simulink model "cst_robotarm_new"  (R2020a)
settings: Solver=ode23t  StartTime=0.0  StopTime=40  FixedStep=0.0001  MaxStep=0.05  RelTol=1e-3  EnableMultiTasking=on
model workspace (MAT data in the model file):
  DCMotor_J = 0.0946866703633
  DCMotor_K = 0.477771340295
  DCMotor_Kf = 0.921434142151
  DCMotor_L = 0.000316454712175
  DCMotor_R = 4.99938152603
  Ts = 0.1
  dFilt = [1 -0.1202]
  nFilt = [0.4399 0.4399]
undefined symbols (not defined in the file): X, Y, Z
libraries: sm_lib x244, fl_lib x75, nesl_utility x28, ee_lib x21
(part 1 of 6)
settings Model: SimulationMode=accelerator  Creator=The MathWorks, Inc.  LastModifiedBy=nikhil
settings DataIOCC: LimitDataPoints=on  SaveFormat=Array  InspectSignalLogs=on  SaveTime=off  ReturnWorkspaceOutputs=off
settings OptimizationCC: ExpressionDepthLimit=2147483647  LifeSpan=inf
settings DebuggingCC: UnderspecifiedInitializationDetection=Classic  MergeDetectMultiDrivingBlocksExec=none  FcnCallInpInsideContextMsg=warning  StateNameClashWarn=warning  SFUnexpectedBacktrackingDiag=warning  SFNoUnconditionalDefaultTransitionDiag=warning  SFExecutionAtInitializationDiag=none  ArithmeticOperatorsInVariantConditions=warning
settings HardwareCC: ProdBitPerPointer=32  ProdBitPerSizeT=32  ProdBitPerPtrDiffT=32  ProdLargestAtomicFloat=None  ProdIntDivRoundTo=Undefined  ProdEndianess=Unspecified  ProdWordSize=32  ProdHWDeviceType=32-bit Generic
settings ModelReferenceCC: PropagateSignalLabelsOutOfModel=off
settings SFSimCC: SimUseLocalCustomCode=off  CustomCodeUndefinedFunction=UseInterfaceOnly
settings RTWCC: RTWUseLocalCustomCode=off
settings CodeAppCC: StateflowObjectComments=on
settings GRTTargetCC: TargetLangStandard=C89/C90 (ANSI)  CombineOutputUpdateFcns=off  GRTInterface=on
settings ConfigComp: CovMetricSettings=dw  CovHtmlReporting=on  CovSaveCumulativeToWorkspaceVar=on  CovSaveSingleToWorkspaceVar=on  CovExternalEMLEnable=off  CovSFcnEnable=off
settings SimscapeCC: SimscapeNormalizeSystem=off
settings ConfigurationSet: Description=SimMechanics 2G
settings DiagnosticsConfigSet: SimMechanicsUnconnectedFramePorts=none
settings ExplorerConfigSet: SimMechanicsOpenEditorOnUpdate=off  InternalSimMechanicsExplorerSettings="<ExplorerConfiguration><canonicalview>planar_xy</canonicalview><AnimationSetting><BasePlaybackSpeed>1.0</BasePlaybackSpeed><PlaybackSpeedFactor>1.0</PlaybackSpeedFactor></AnimationSetting><TilePanel><TileInfo><Tiles Columns=\"1\" Count=\"1\" Rows=\"1\"><Column Left=\"2\" Weight=\"1\"/><Column Left=\"708\"/><Row Top=\"2\" Weight=\"1\"/><Row Top=\"595\"/><Tile Height=\"1\" Width=\"1\" X=\"0\" Y=\"0\"/></Tiles></TileInfo><SceneInfo><SceneViewer><BGColor><R>0.80000001192092896</R><G>0.80000001192092896</G><B>0.80000001192092896</B></BGColor><Camera><Position><X>0.30752487944302698</X><Y>0.57922836563106395</Y><Z>0.35651305744246536</Z></Position><Center><X>-0.033772386749033274</X><Y>0.23793109943898419</Y><Z>0.015215791250393121</Z></Center><Up><X>-0.40824829046386307</X><Y>0.81649658092772615</Y><Z>-0.40824829046386307</Z></Up><Left>-0.063283674940751766</Left><Right>0.063283674940751766</Right><Bottom>-0.22321517040744418</Bottom><Top>0.22321517040744418</Top></Camera></SceneViewer></SceneInfo></TilePanel></ExplorerConfiguration>"

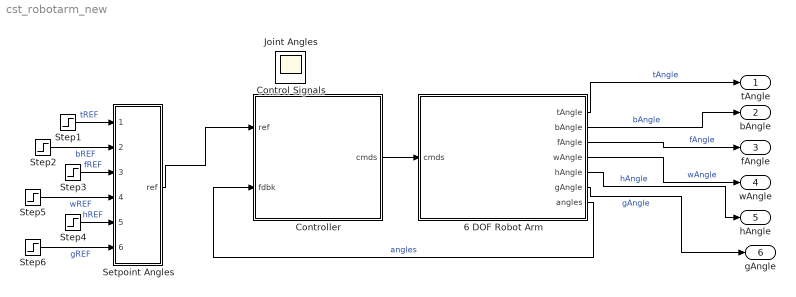
== system cst_robotarm_new ==
  6 DOF Robot Arm : Subsystem
      mask Display: image('RobotArmSystem.jpg',[0.2 0.05 0.6 0.9])
  Controller : Subsystem
  Setpoint Angles : Subsystem
  Step1 : Step  Time=0  After=60  SampleTime=Ts
  Step2 : Step  Time=0  Before=90  After=80  SampleTime=Ts
  Step3 : Step  Time=0  After=60  SampleTime=Ts
  Step4 : Step  Time=0  After=90  SampleTime=Ts
  Step5 : Step  Time=0  After=90  SampleTime=Ts
  Step6 : Step  Time=0  After=60  SampleTime=Ts
  tAngle : Outport
  bAngle : Outport  Port=2
  fAngle : Outport  Port=3
  wAngle : Outport  Port=4
  hAngle : Outport  Port=5
  gAngle : Outport  Port=6
  Control Signals : Scope
  Joint Angles : Scope
  wires:
  Controller/1(cmds) -> 6 DOF Robot Arm/1(cmds)
  6 DOF Robot Arm/7(angles) -> Controller/2(fdbk)  "angles"
  Setpoint Angles/1(ref) -> Controller/1(ref)
  Step2/1 -> Setpoint Angles/2(bREF)  "bREF"
  Step1/1 -> Setpoint Angles/1(tREF)  "tREF"
  Step4/1 -> Setpoint Angles/5(hREF)  "hREF"
  Step5/1 -> Setpoint Angles/4(wREF)  "wREF"
  Step3/1 -> Setpoint Angles/3(fREF)  "fREF"
  Step6/1 -> Setpoint Angles/6(gREF)  "gREF"
  6 DOF Robot Arm/1(tAngle) -> tAngle/1  "tAngle"
  6 DOF Robot Arm/2(bAngle) -> bAngle/1  "bAngle"
  6 DOF Robot Arm/3(fAngle) -> fAngle/1  "fAngle"
  6 DOF Robot Arm/4(wAngle) -> wAngle/1  "wAngle"
  6 DOF Robot Arm/5(hAngle) -> hAngle/1  "hAngle"
  6 DOF Robot Arm/6(gAngle) -> gAngle/1  "gAngle"

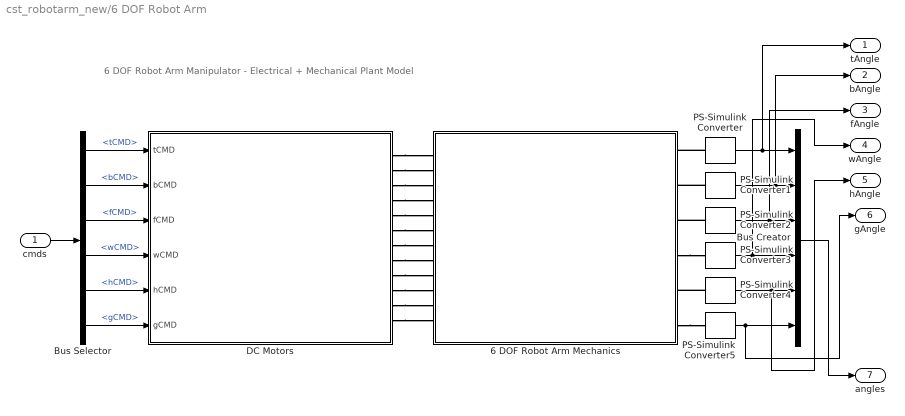
== system cst_robotarm_new/6 DOF Robot Arm ==
  note: 6 DOF Robot Arm Manipulator - Electrical + Mechanical Plant Model
  cmds : Inport
  6 DOF Robot Arm Mechanics : Subsystem
      mask Display: image('RobotArm_Mechanics.jpg',[0.1 0 0.8 1])
  Bus Creator : BusCreator  Inputs=6
  Bus Selector : BusSelector  OutputSignals=tCMD,bCMD,fCMD,wCMD,hCMD,gCMD
  DC Motors : Subsystem
      mask Display: image('MultiServos.jpg',[0.25 0.1 0.5 0.8])
  PS-Simulink Converter{,1..5} (6 alike) : nesl_utility/PS-Simulink Converter  PhysicalDomain=network_engine_domain  SubClassName=ps_output  LeftPortType=input  RightPortType=output  PseudoPeriodic=off  Frequencies=[]  Unit=rad  AffineConversion=off
      settings: SourceProductBaseCode=MT,SS
  tAngle : Outport
  bAngle : Outport  Port=2
  fAngle : Outport  Port=3
  wAngle : Outport  Port=4
  hAngle : Outport  Port=5
  gAngle : Outport  Port=6
  angles : Outport  Port=7  VectorParamsAs1DForOutWhenUnconnected=off
  wires:
  Bus Creator/1 -> angles/1
  PS-Simulink Converter2/1 -> fAngle/1, Bus Creator/3
  PS-Simulink Converter5/1 -> gAngle/1, Bus Creator/6
  PS-Simulink Converter/1 -> tAngle/1, Bus Creator/1
  PS-Simulink Converter1/1 -> bAngle/1, Bus Creator/2
  PS-Simulink Converter3/1 -> wAngle/1, Bus Creator/4
  PS-Simulink Converter4/1 -> hAngle/1, Bus Creator/5
  Bus Selector/6 -> DC Motors/6(gCMD)  "<gCMD>"
  Bus Selector/3 -> DC Motors/3(fCMD)  "<fCMD>"
  Bus Selector/4 -> DC Motors/4(wCMD)  "<wCMD>"
  Bus Selector/2 -> DC Motors/2(bCMD)  "<bCMD>"
  Bus Selector/5 -> DC Motors/5(hCMD)  "<hCMD>"
  Bus Selector/1 -> DC Motors/1(tCMD)  "<tCMD>"
  cmds/1 -> Bus Selector/1
  connections:
  PS-Simulink Converter2/LConn1 -- 6 DOF Robot Arm Mechanics/RConn3
  DC Motors/RConn7 -- 6 DOF Robot Arm Mechanics/LConn7
  DC Motors/RConn8 -- 6 DOF Robot Arm Mechanics/LConn8
  DC Motors/RConn6 -- 6 DOF Robot Arm Mechanics/LConn6
  PS-Simulink Converter/LConn1 -- 6 DOF Robot Arm Mechanics/RConn1
  DC Motors/RConn2 -- 6 DOF Robot Arm Mechanics/LConn2
  DC Motors/RConn5 -- 6 DOF Robot Arm Mechanics/LConn5
  DC Motors/RConn11 -- 6 DOF Robot Arm Mechanics/LConn11
  DC Motors/RConn12 -- 6 DOF Robot Arm Mechanics/LConn12
  DC Motors/RConn9 -- 6 DOF Robot Arm Mechanics/LConn9
  DC Motors/RConn3 -- 6 DOF Robot Arm Mechanics/LConn3
  DC Motors/RConn4 -- 6 DOF Robot Arm Mechanics/LConn4
  PS-Simulink Converter1/LConn1 -- 6 DOF Robot Arm Mechanics/RConn2
  PS-Simulink Converter4/LConn1 -- 6 DOF Robot Arm Mechanics/RConn5
  6 DOF Robot Arm Mechanics/RConn6 -- PS-Simulink Converter5/LConn1
  6 DOF Robot Arm Mechanics/RConn4 -- PS-Simulink Converter3/LConn1
  DC Motors/RConn10 -- 6 DOF Robot Arm Mechanics/LConn10
  DC Motors/RConn1 -- 6 DOF Robot Arm Mechanics/LConn1

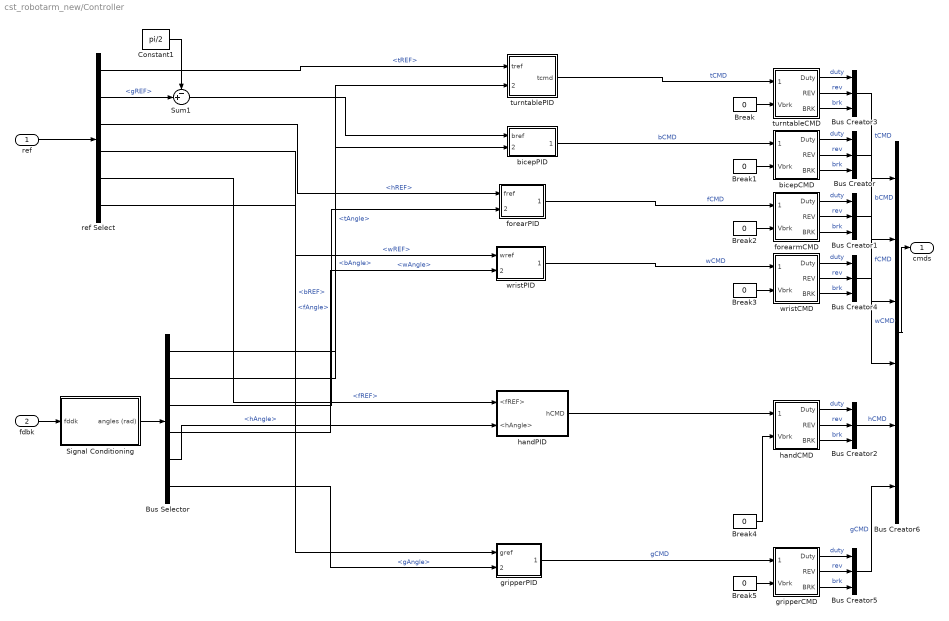
== system cst_robotarm_new/Controller ==
  ref : Inport
  fdbk : Inport  Port=2
  Break{,1..5} (6 alike) : Constant  Value=0
  Bus Creator{,1..5} (6 alike) : BusCreator  Inputs=3
  Bus Creator6 : BusCreator  Inputs=6
  Bus Selector : BusSelector  OutputSignals=tAngle,bAngle,fAngle,wAngle,hAngle,gAngle
  Constant1 : Constant  Value=pi/2
  Signal Conditioning : Subsystem
  Sum1 : Sum  Inputs=-+|
  bicepCMD : Subsystem
  bicepPID : Subsystem
  forearPID : Subsystem
  forearmCMD : Subsystem
  gripperCMD : Subsystem
  gripperPID : Subsystem
  handCMD : Subsystem
  handPID : Subsystem
  ref Select : BusSelector  OutputSignals=tREF,gREF,hREF,wREF,fREF,bREF
  turntableCMD : Subsystem
  turntablePID : Subsystem
  wristCMD : Subsystem
  wristPID : Subsystem
  cmds : Outport  VectorParamsAs1DForOutWhenUnconnected=off
  wires:
  bicepCMD/1(Duty) -> Bus Creator/1  "duty"
  bicepCMD/2(REV) -> Bus Creator/2  "rev"
  bicepCMD/3(BRK) -> Bus Creator/3  "brk"
  forearmCMD/1(Duty) -> Bus Creator1/1  "duty"
  forearmCMD/2(REV) -> Bus Creator1/2  "rev"
  forearmCMD/3(BRK) -> Bus Creator1/3  "brk"
  handCMD/2(REV) -> Bus Creator2/2  "rev"
  handCMD/3(BRK) -> Bus Creator2/3  "brk"
  handCMD/1(Duty) -> Bus Creator2/1  "duty"
  bicepPID/1(bcmd) -> bicepCMD/1(Vcmd)  "bCMD"
  Break1/1 -> bicepCMD/2(Vbrk)
  forearPID/1(fcmd) -> forearmCMD/1(Vcmd)  "fCMD"
  Break2/1 -> forearmCMD/2(Vbrk)
  Break4/1 -> handCMD/2(Vbrk)
  Bus Creator1/1 -> Bus Creator6/3  "fCMD"
  Bus Creator2/1 -> Bus Creator6/5  "hCMD"
  ref/1 -> ref Select/1
  turntableCMD/1(Duty) -> Bus Creator3/1  "duty"
  turntableCMD/2(REV) -> Bus Creator3/2  "rev"
  turntableCMD/3(BRK) -> Bus Creator3/3  "brk"
  turntablePID/1(tcmd) -> turntableCMD/1(Vcmd)  "tCMD"
  Break/1 -> turntableCMD/2(Vbrk)
  Bus Creator3/1 -> Bus Creator6/1  "tCMD"
  wristCMD/2(REV) -> Bus Creator4/2  "rev"
  wristCMD/3(BRK) -> Bus Creator4/3  "brk"
  wristCMD/1(Duty) -> Bus Creator4/1  "duty"
  wristPID/1(wcmd) -> wristCMD/1(Vcmd)  "wCMD"
  Break3/1 -> wristCMD/2(Vbrk)
  Bus Creator4/1 -> Bus Creator6/4  "wCMD"
  gripperCMD/2(REV) -> Bus Creator5/2  "rev"
  gripperCMD/3(BRK) -> Bus Creator5/3  "brk"
  gripperCMD/1(Duty) -> Bus Creator5/1  "duty"
  gripperPID/1(gcmd) -> gripperCMD/1(Vcmd)  "gCMD"
  Break5/1 -> gripperCMD/2(Vbrk)
  Bus Creator5/1 -> Bus Creator6/6  "gCMD"
  Bus Creator/1 -> Bus Creator6/2  "bCMD"
  Bus Creator6/1 -> cmds/1
  Bus Selector/6 -> gripperPID/2(gangle)  "<gAngle>"
  Bus Selector/5 -> handPID/2(<hAngle>)  "<hAngle>"
  Bus Selector/4 -> wristPID/2(wangle)  "<wAngle>"
  Bus Selector/3 -> forearPID/2(fangle)  "<fAngle>"
  Bus Selector/1 -> turntablePID/2(tangle)  "<tAngle>"
  ref Select/1 -> turntablePID/1(tref)  "<tREF>"
  ref Select/3 -> forearPID/1(fref)  "<hREF>"
  ref Select/4 -> wristPID/1(wref)  "<wREF>"
  ref Select/6 -> gripperPID/1(gref)  "<bREF>"
  fdbk/1 -> Signal Conditioning/1(fddk)
  Signal Conditioning/1(angles (rad)) -> Bus Selector/1
  Sum1/1 -> bicepPID/1(bref)
  ref Select/2 -> Sum1/2  "<gREF>"
  Constant1/1 -> Sum1/1
  Bus Selector/2 -> bicepPID/2(bangle)  "<bAngle>"
  ref Select/5 -> handPID/1(<fREF>)  "<fREF>"
  handPID/1(hCMD) -> handCMD/1(Vcmd)

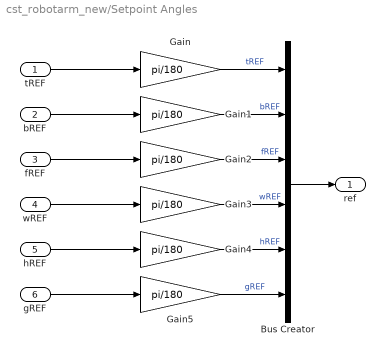
== system cst_robotarm_new/Setpoint Angles ==
  tREF : Inport
  bREF : Inport  Port=2
  fREF : Inport  Port=3
  wREF : Inport  Port=4
  hREF : Inport  Port=5
  gREF : Inport  Port=6
  Bus Creator : BusCreator  Inputs=6
  Gain{,1..5} (6 alike) : Gain  Gain=pi/180
  ref : Outport  VectorParamsAs1DForOutWhenUnconnected=off
  wires:
  Gain5/1 -> Bus Creator/6  "gREF"
  fREF/1 -> Gain2/1
  Gain4/1 -> Bus Creator/5  "hREF"
  bREF/1 -> Gain1/1
  tREF/1 -> Gain/1
  Bus Creator/1 -> ref/1
  Gain3/1 -> Bus Creator/4  "wREF"
  Gain1/1 -> Bus Creator/2  "bREF"
  Gain/1 -> Bus Creator/1  "tREF"
  Gain2/1 -> Bus Creator/3  "fREF"
  wREF/1 -> Gain3/1
  hREF/1 -> Gain4/1
  gREF/1 -> Gain5/1

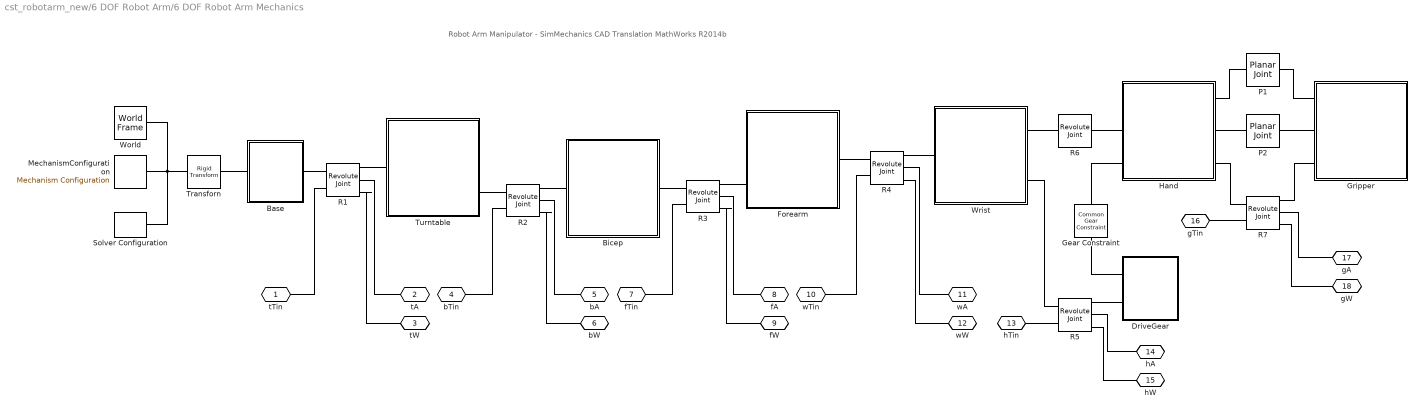
== system cst_robotarm_new/6 DOF Robot Arm/6 DOF Robot Arm Mechanics ==
  note: Robot Arm Manipulator - SimMechanics CAD Translation
      | MathWorks R2014b
  Base : Subsystem
      mask Display: image('Base.jpg',[0.25,0.25,0.5,0.5])
  Bicep : Subsystem
      mask Display: image('Bicep.jpg')
  DriveGear : Subsystem
      mask Display: image('DriveGear.jpg',[0.2,0.2,0.6,0.6])
  Forearm : Subsystem
      mask Display: image('Forearm.jpg')
  Gear Constraint : sm_lib/Gears and Couplings/Gears/Common Gear Constraint  GearType=External  SpecificationType=CenterDistanceRatio  CenterDistance=39.8888296  CenterDistanceUnits=mm  GearRatio=1.0  BaseGearRadius=10.0  BaseGearRadiusUnits=cm  FollGearRadius=10.0  FollGearRadiusUnits=cm  AssemblyGearRotation=Free
      settings: SourceProductBaseCode=MS
  Gripper : Subsystem
      mask Display: image('Gripper.jpg',[0.1,0.1,0.8,0.8])
  Hand : Subsystem
      mask Display: image('Hand.jpg',[0.1,0.1,0.8,0.8])
  MechanismConfiguration : sm_lib/Utilities/Mechanism Configuration  UniformGravity=Constant  GravityVector=[0 -9.81 0]  GravityUnits=m/s^2  LinearizationDelta=0.001
  P1 : sm_lib/Joints/Planar Joint  JointMode=Normal  SenseConstraintForce=off  SenseConstraintForceX=off  SenseConstraintForceY=off  SenseConstraintForceZ=off  SenseConstraintTorque=off  SenseConstraintTorqueX=off  SenseConstraintTorqueY=off  SenseConstraintTorqueZ=off  SenseTotalForce=off  SenseTotalForceX=off  SenseTotalForceY=off  SenseTotalForceZ=off  SenseTotalTorque=off  SenseTotalTorqueX=off  SenseTotalTorqueY=off  SenseTotalTorqueZ=off  CompositeWrenchDir=FollowerOnBase  CompositeWrenchFrame=BaseFrame  PxEquilibriumPosition=0  PxEquilibriumPositionUnits=m  PxSpringStiffness=0  PxSpringStiffnessUnits=N/m  PxDampingCoefficient=0  PxDampingCoefficientUnits=s*N/m  PxTorqueActuationMode=NoTorque  PxMotionActuationMode=ComputedMotion  PxSensePosition=off  PxSenseVelocity=off  PxSenseAcceleration=off  PxSenseTorqueForce=off  PxSenseLowerLimitTorqueForce=off  PxSenseUpperLimitTorqueForce=off  PxLowerLimitSpecify=off  PxLowerLimitBound=-1  PxLowerLimitBoundUnits=m  PxLowerLimitStiffness=1e6  PxLowerLimitStiffnessUnits=N/m  PxLowerLimitDamping=1e3  PxLowerLimitDampingUnits=N/(m/s)  PxLowerLimitTransitionRegionWidth=1e-4  PxLowerLimitTransitionRegionWidthUnits=m  PxUpperLimitSpecify=off  PxUpperLimitBound=1  PxUpperLimitBoundUnits=m  PxUpperLimitStiffness=1e6  PxUpperLimitStiffnessUnits=N/m  PxUpperLimitDamping=1e3  PxUpperLimitDampingUnits=N/(m/s)  PxUpperLimitTransitionRegionWidth=1e-4  PxUpperLimitTransitionRegionWidthUnits=m  PxPositionTargetSpecify=off  PxPositionTargetPriority=High  PxPositionTargetValue=0  PxPositionTargetValueUnits=m  PxVelocityTargetSpecify=off  PxVelocityTargetPriority=High  PxVelocityTargetValue=0  PxVelocityTargetValueUnits=m/s  PyEquilibriumPosition=0  PyEquilibriumPositionUnits=m  PySpringStiffness=0  PySpringStiffnessUnits=N/m  PyDampingCoefficient=0  PyDampingCoefficientUnits=s*N/m  PyTorqueActuationMode=NoTorque  PyMotionActuationMode=ComputedMotion  PySensePosition=off  PySenseVelocity=off  PySenseAcceleration=off  PySenseTorqueForce=off  PySenseLowerLimitTorqueForce=off  PySenseUpperLimitTorqueForce=off  PyLowerLimitSpecify=off  PyLowerLimitBound=-1  PyLowerLimitBoundUnits=m  PyLowerLimitStiffness=1e6  PyLowerLimitStiffnessUnits=N/m  PyLowerLimitDamping=1e3  PyLowerLimitDampingUnits=N/(m/s)  PyLowerLimitTransitionRegionWidth=1e-4  PyLowerLimitTransitionRegionWidthUnits=m  PyUpperLimitSpecify=off  PyUpperLimitBound=1  PyUpperLimitBoundUnits=m  PyUpperLimitStiffness=1e6  PyUpperLimitStiffnessUnits=N/m  PyUpperLimitDamping=1e3  PyUpperLimitDampingUnits=N/(m/s)  PyUpperLimitTransitionRegionWidth=1e-4  PyUpperLimitTransitionRegionWidthUnits=m  PyPositionTargetSpecify=off  PyPositionTargetPriority=High  PyPositionTargetValue=0  PyPositionTargetValueUnits=m  PyVelocityTargetSpecify=off  PyVelocityTargetPriority=High  PyVelocityTargetValue=0  PyVelocityTargetValueUnits=m/s  RzEquilibriumPosition=0  RzEquilibriumPositionUnits=rad  RzSpringStiffness=0  RzSpringStiffnessUnits=m*N/rad  RzDampingCoefficient=0  RzDampingCoefficientUnits=m*s*N/rad  RzTorqueActuationMode=NoTorque  RzMotionActuationMode=ComputedMotion  RzSensePosition=off  RzSenseVelocity=off  RzSenseAcceleration=off  RzSenseTorqueForce=off  RzSenseLowerLimitTorqueForce=off  RzSenseUpperLimitTorqueForce=off  RzLowerLimitSpecify=off  RzLowerLimitBound=-90  RzLowerLimitBoundUnits=deg  RzLowerLimitStiffness=1e4  RzLowerLimitStiffnessUnits=N*m/deg  RzLowerLimitDamping=10  RzLowerLimitDampingUnits=N*m/(deg/s)  RzLowerLimitTransitionRegionWidth=0.1  RzLowerLimitTransitionRegionWidthUnits=deg  RzUpperLimitSpecify=off  RzUpperLimitBound=90  RzUpperLimitBoundUnits=deg  RzUpperLimitStiffness=1e4  RzUpperLimitStiffnessUnits=N*m/deg  RzUpperLimitDamping=10  RzUpperLimitDampingUnits=N*m/(deg/s)  RzUpperLimitTransitionRegionWidth=0.1  RzUpperLimitTransitionRegionWidthUnits=deg  RzPositionTargetSpecify=off  RzPositionTargetPriority=High  RzPositionTargetValue=0  RzPositionTargetValueUnits=deg  RzVelocityTargetSpecify=off  RzVelocityTargetPriority=High  RzVelocityTargetValue=0  RzVelocityTargetValueUnits=deg/s
  P2 : sm_lib/Joints/Planar Joint  JointMode=Normal  SenseConstraintForce=off  SenseConstraintForceX=off  SenseConstraintForceY=off  SenseConstraintForceZ=off  SenseConstraintTorque=off  SenseConstraintTorqueX=off  SenseConstraintTorqueY=off  SenseConstraintTorqueZ=off  SenseTotalForce=off  SenseTotalForceX=off  SenseTotalForceY=off  SenseTotalForceZ=off  SenseTotalTorque=off  SenseTotalTorqueX=off  SenseTotalTorqueY=off  SenseTotalTorqueZ=off  CompositeWrenchDir=FollowerOnBase  CompositeWrenchFrame=BaseFrame  PxEquilibriumPosition=0  PxEquilibriumPositionUnits=m  PxSpringStiffness=0  PxSpringStiffnessUnits=N/m  PxDampingCoefficient=0  PxDampingCoefficientUnits=s*N/m  PxTorqueActuationMode=NoTorque  PxMotionActuationMode=ComputedMotion  PxSensePosition=off  PxSenseVelocity=off  PxSenseAcceleration=off  PxSenseTorqueForce=off  PxSenseLowerLimitTorqueForce=off  PxSenseUpperLimitTorqueForce=off  PxLowerLimitSpecify=off  PxLowerLimitBound=-1  PxLowerLimitBoundUnits=m  PxLowerLimitStiffness=1e6  PxLowerLimitStiffnessUnits=N/m  PxLowerLimitDamping=1e3  PxLowerLimitDampingUnits=N/(m/s)  PxLowerLimitTransitionRegionWidth=1e-4  PxLowerLimitTransitionRegionWidthUnits=m  PxUpperLimitSpecify=off  PxUpperLimitBound=1  PxUpperLimitBoundUnits=m  PxUpperLimitStiffness=1e6  PxUpperLimitStiffnessUnits=N/m  PxUpperLimitDamping=1e3  PxUpperLimitDampingUnits=N/(m/s)  PxUpperLimitTransitionRegionWidth=1e-4  PxUpperLimitTransitionRegionWidthUnits=m  PxPositionTargetSpecify=off  PxPositionTargetPriority=High  PxPositionTargetValue=0  PxPositionTargetValueUnits=m  PxVelocityTargetSpecify=off  PxVelocityTargetPriority=High  PxVelocityTargetValue=0  PxVelocityTargetValueUnits=m/s  PyEquilibriumPosition=0  PyEquilibriumPositionUnits=m  PySpringStiffness=0  PySpringStiffnessUnits=N/m  PyDampingCoefficient=0  PyDampingCoefficientUnits=s*N/m  PyTorqueActuationMode=NoTorque  PyMotionActuationMode=ComputedMotion  PySensePosition=off  PySenseVelocity=off  PySenseAcceleration=off  PySenseTorqueForce=off  PySenseLowerLimitTorqueForce=off  PySenseUpperLimitTorqueForce=off  PyLowerLimitSpecify=off  PyLowerLimitBound=-1  PyLowerLimitBoundUnits=m  PyLowerLimitStiffness=1e6  PyLowerLimitStiffnessUnits=N/m  PyLowerLimitDamping=1e3  PyLowerLimitDampingUnits=N/(m/s)  PyLowerLimitTransitionRegionWidth=1e-4  PyLowerLimitTransitionRegionWidthUnits=m  PyUpperLimitSpecify=off  PyUpperLimitBound=1  PyUpperLimitBoundUnits=m  PyUpperLimitStiffness=1e6  PyUpperLimitStiffnessUnits=N/m  PyUpperLimitDamping=1e3  PyUpperLimitDampingUnits=N/(m/s)  PyUpperLimitTransitionRegionWidth=1e-4  PyUpperLimitTransitionRegionWidthUnits=m  PyPositionTargetSpecify=off  PyPositionTargetPriority=High  PyPositionTargetValue=0  PyPositionTargetValueUnits=m  PyVelocityTargetSpecify=off  PyVelocityTargetPriority=High  PyVelocityTargetValue=0  PyVelocityTargetValueUnits=m/s  RzEquilibriumPosition=0  RzEquilibriumPositionUnits=rad  RzSpringStiffness=0  RzSpringStiffnessUnits=m*N/rad  RzDampingCoefficient=0  RzDampingCoefficientUnits=m*s*N/rad  RzTorqueActuationMode=NoTorque  RzMotionActuationMode=ComputedMotion  RzSensePosition=off  RzSenseVelocity=off  RzSenseAcceleration=off  RzSenseTorqueForce=off  RzSenseLowerLimitTorqueForce=off  RzSenseUpperLimitTorqueForce=off  RzLowerLimitSpecify=off  RzLowerLimitBound=-90  RzLowerLimitBoundUnits=deg  RzLowerLimitStiffness=1e4  RzLowerLimitStiffnessUnits=N*m/deg  RzLowerLimitDamping=10  RzLowerLimitDampingUnits=N*m/(deg/s)  RzLowerLimitTransitionRegionWidth=0.1  RzLowerLimitTransitionRegionWidthUnits=deg  RzUpperLimitSpecify=off  RzUpperLimitBound=90  RzUpperLimitBoundUnits=deg  RzUpperLimitStiffness=1e4  RzUpperLimitStiffnessUnits=N*m/deg  RzUpperLimitDamping=10  RzUpperLimitDampingUnits=N*m/(deg/s)  RzUpperLimitTransitionRegionWidth=0.1  RzUpperLimitTransitionRegionWidthUnits=deg  RzPositionTargetSpecify=off  RzPositionTargetPriority=High  RzPositionTargetValue=0  RzPositionTargetValueUnits=deg  RzVelocityTargetSpecify=off  RzVelocityTargetPriority=High  RzVelocityTargetValue=0  RzVelocityTargetValueUnits=deg/s
  R{1,3..5,7} (5 alike) : sm_lib/Joints/Revolute Joint  JointMode=Normal  SenseConstraintForce=off  SenseConstraintForceX=off  SenseConstraintForceY=off  SenseConstraintForceZ=off  SenseConstraintTorque=off  SenseConstraintTorqueX=off  SenseConstraintTorqueY=off  SenseConstraintTorqueZ=off  SenseTotalForce=off  SenseTotalForceX=off  SenseTotalForceY=off  SenseTotalForceZ=off  SenseTotalTorque=off  SenseTotalTorqueX=off  SenseTotalTorqueY=off  SenseTotalTorqueZ=off  CompositeWrenchDir=FollowerOnBase  CompositeWrenchFrame=BaseFrame  EquilibriumPosition=0  EquilibriumPositionUnits=rad  SpringStiffness=0  SpringStiffnessUnits=m*N/rad  DampingCoefficient=0  DampingCoefficientUnits=m*s*N/rad  TorqueActuationMode=InputTorque  MotionActuationMode=ComputedMotion  SensePosition=on  SenseVelocity=on  SenseAcceleration=off  SenseTorqueForce=off  SenseLowerLimitTorqueForce=off  SenseUpperLimitTorqueForce=off  LowerLimitSpecify=off  LowerLimitBound=-90  LowerLimitBoundUnits=deg  LowerLimitStiffness=1e4  LowerLimitStiffnessUnits=N*m/deg  LowerLimitDamping=10  LowerLimitDampingUnits=N*m/(deg/s)  LowerLimitTransitionRegionWidth=0.1  LowerLimitTransitionRegionWidthUnits=deg  UpperLimitSpecify=off  UpperLimitBound=90  UpperLimitBoundUnits=deg  UpperLimitStiffness=1e4  UpperLimitStiffnessUnits=N*m/deg  UpperLimitDamping=10  UpperLimitDampingUnits=N*m/(deg/s)  UpperLimitTransitionRegionWidth=0.1  UpperLimitTransitionRegionWidthUnits=deg  PositionTargetSpecify=on  PositionTargetPriority=High  PositionTargetValue=0  PositionTargetValueUnits=deg  VelocityTargetSpecify=on  VelocityTargetPriority=High  VelocityTargetValue=0  VelocityTargetValueUnits=deg/s
  R2 : sm_lib/Joints/Revolute Joint  JointMode=Normal  SenseConstraintForce=off  SenseConstraintForceX=off  SenseConstraintForceY=off  SenseConstraintForceZ=off  SenseConstraintTorque=off  SenseConstraintTorqueX=off  SenseConstraintTorqueY=off  SenseConstraintTorqueZ=off  SenseTotalForce=off  SenseTotalForceX=off  SenseTotalForceY=off  SenseTotalForceZ=off  SenseTotalTorque=off  SenseTotalTorqueX=off  SenseTotalTorqueY=off  SenseTotalTorqueZ=off  CompositeWrenchDir=FollowerOnBase  CompositeWrenchFrame=BaseFrame  EquilibriumPosition=0  EquilibriumPositionUnits=rad  SpringStiffness=0  SpringStiffnessUnits=m*N/rad  DampingCoefficient=0  DampingCoefficientUnits=m*s*N/rad  TorqueActuationMode=InputTorque  MotionActuationMode=ComputedMotion  SensePosition=on  SenseVelocity=on  SenseAcceleration=off  SenseTorqueForce=off  SenseLowerLimitTorqueForce=off  SenseUpperLimitTorqueForce=off  LowerLimitSpecify=off  LowerLimitBound=-90  LowerLimitBoundUnits=deg  LowerLimitStiffness=1e4  LowerLimitStiffnessUnits=N*m/deg  LowerLimitDamping=10  LowerLimitDampingUnits=N*m/(deg/s)  LowerLimitTransitionRegionWidth=0.1  LowerLimitTransitionRegionWidthUnits=deg  UpperLimitSpecify=off  UpperLimitBound=90  UpperLimitBoundUnits=deg  UpperLimitStiffness=1e4  UpperLimitStiffnessUnits=N*m/deg  UpperLimitDamping=10  UpperLimitDampingUnits=N*m/(deg/s)  UpperLimitTransitionRegionWidth=0.1  UpperLimitTransitionRegionWidthUnits=deg  PositionTargetSpecify=on  PositionTargetPriority=High  PositionTargetValue=90  PositionTargetValueUnits=deg  VelocityTargetSpecify=on  VelocityTargetPriority=High  VelocityTargetValue=0  VelocityTargetValueUnits=deg/s
  R6 : sm_lib/Joints/Revolute Joint  JointMode=Normal  SenseConstraintForce=off  SenseConstraintForceX=off  SenseConstraintForceY=off  SenseConstraintForceZ=off  SenseConstraintTorque=off  SenseConstraintTorqueX=off  SenseConstraintTorqueY=off  SenseConstraintTorqueZ=off  SenseTotalForce=off  SenseTotalForceX=off  SenseTotalForceY=off  SenseTotalForceZ=off  SenseTotalTorque=off  SenseTotalTorqueX=off  SenseTotalTorqueY=off  SenseTotalTorqueZ=off  CompositeWrenchDir=FollowerOnBase  CompositeWrenchFrame=BaseFrame  EquilibriumPosition=0  EquilibriumPositionUnits=rad  SpringStiffness=0  SpringStiffnessUnits=m*N/rad  DampingCoefficient=0  DampingCoefficientUnits=m*s*N/rad  TorqueActuationMode=NoTorque  MotionActuationMode=ComputedMotion  SensePosition=off  SenseVelocity=off  SenseAcceleration=off  SenseTorqueForce=off  SenseLowerLimitTorqueForce=off  SenseUpperLimitTorqueForce=off  LowerLimitSpecify=off  LowerLimitBound=-90  LowerLimitBoundUnits=deg  LowerLimitStiffness=1e4  LowerLimitStiffnessUnits=N*m/deg  LowerLimitDamping=10  LowerLimitDampingUnits=N*m/(deg/s)  LowerLimitTransitionRegionWidth=0.1  LowerLimitTransitionRegionWidthUnits=deg  UpperLimitSpecify=off  UpperLimitBound=90  UpperLimitBoundUnits=deg  UpperLimitStiffness=1e4  UpperLimitStiffnessUnits=N*m/deg  UpperLimitDamping=10  UpperLimitDampingUnits=N*m/(deg/s)  UpperLimitTransitionRegionWidth=0.1  UpperLimitTransitionRegionWidthUnits=deg  PositionTargetSpecify=on  PositionTargetPriority=High  PositionTargetValue=-90  PositionTargetValueUnits=deg  VelocityTargetSpecify=on  VelocityTargetPriority=High  VelocityTargetValue=0  VelocityTargetValueUnits=deg/s
  Solver Configuration : nesl_utility/Solver Configuration  PhysicalDomain=network_engine_domain  SubClassName=solver  LeftPortType=input  RightPortType=generic  Tones=[]  Harmonics=[]  SimulateNoise=off  Profile=off  UseLocalSampling=off  EnableSwitchedLinearOptims=on  FrequencyDomain=off  UseCCode=off  RelTol=0.001  AbsTol=1e-06  MinStep=1e-09  ToWorkspace=off  RevertToSquareIcSolve=off  NumHomotopyIterations=100  PhasorMode=off  PhasorModeNumHarmonics=1  DoDC=off  ResidualTolerance=1e-09  UseLocalSolver=off  LocalSolverChoice=NE_BACKWARD_EULER_ADVANCER  LocalSolverSampleTime=0.001  DoFixedCost=off  MaxNonlinIter=3  MaxModeIter=2  LinearAlgebra=Sparse  EquationFormulation=NE_TIME_EF  DelaysMemoryBudget=1024  AutomaticFiltering=on  FilteringTimeConstant=0.001  PartitionStorageMethod=AS_NEEDED  PartitionMemoryBudget=1024  PartitionMethod=FAST
      settings: SourceProductBaseCode=MT,SS
  Transforn : sm_lib/Frames and Transforms/Rigid Transform  TranslationMethod=None  TranslationStandardOffset=0  TranslationLengthUnit=m  TranslationStandardAxis=+Z  TranslationCartesianOffset=[0 0 0]  TranslationROffset=0  TranslationROffsetUnits=m  TranslationZOffset=0  TranslationZOffsetUnits=m  TranslationThetaOffset=0  TranslationThetaOffsetUnits=deg  RotationMethod=None  RotationAngleUnits=deg  RotationStandardAxis=+Z  RotationAngle=0.0  RotationArbitraryAxis=[0 0 1]  FollAlignAxisA=+X  BaseAlignAxisA=+Y  FollAlignAxisB=+Y  BaseAlignAxisB=+Z  RotationSequenceAxes=FollowerAxes  RotationSequence=XYX  RotationSequenceAngles=[0 0 0]  RotationSequenceAnglesUnits=deg  RotationMatrix=[1 0 0; 0 1 0; 0 0 1]
  Turntable : Subsystem
      mask Display: image('Turntable.jpg')
  World : sm_lib/Frames and Transforms/World Frame
  Wrist : Subsystem
      mask Display: image('Wrist.jpg')
  tTin : PMIOPort  Side=Left
  tA : PMIOPort  Port=2  Side=Right
  tW : PMIOPort  Port=3  Side=Left
  bTin : PMIOPort  Port=4  Side=Left
  bA : PMIOPort  Port=5  Side=Right
  bW : PMIOPort  Port=6  Side=Left
  fTin : PMIOPort  Port=7  Side=Left
  fA : PMIOPort  Port=8  Side=Right
  fW : PMIOPort  Port=9  Side=Left
  wTin : PMIOPort  Port=10  Side=Left
  wA : PMIOPort  Port=11  Side=Right
  wW : PMIOPort  Port=12  Side=Left
  hTin : PMIOPort  Port=13  Side=Left
  hA : PMIOPort  Port=14  Side=Right
  hW : PMIOPort  Port=15  Side=Left
  gTin : PMIOPort  Port=16  Side=Left
  gA : PMIOPort  Port=17  Side=Right
  gW : PMIOPort  Port=18  Side=Left
  connections:
  World/RConn1 -- Transforn/LConn1 -- MechanismConfiguration/RConn1 -- Solver Configuration/RConn1
  R2/LConn1 -- Turntable/RConn2
  Gripper/LConn3 -- R7/RConn1
  Hand/RConn2 -- P2/LConn1
  Gripper/LConn2 -- P2/RConn1
  R6/LConn1 -- Wrist/RConn1
  Hand/LConn2 -- R6/RConn1
  Hand/RConn1 -- P1/LConn1
  Gripper/LConn1 -- P1/RConn1
  Forearm/RConn1 -- R4/LConn1
  R4/RConn1 -- Wrist/LConn1
  Base/LConn1 -- Transforn/RConn1
  Bicep/LConn1 -- R2/RConn1
  Bicep/RConn1 -- R3/LConn1
  Forearm/LConn2 -- R3/RConn1
  R5/LConn1 -- Wrist/RConn2
  DriveGear/LConn2 -- R5/RConn1
  Base/RConn1 -- R1/LConn1
  R1/RConn1 -- Turntable/LConn1
  Hand/RConn3 -- R7/LConn1
  tTin/RConn1 -- R1/LConn2
  bTin/RConn1 -- R2/LConn2
  fTin/RConn1 -- R3/LConn2
  wTin/RConn1 -- R4/LConn2
  hTin/RConn1 -- R5/LConn2
  gTin/RConn1 -- R7/LConn2
  Gear Constraint/LConn1 -- DriveGear/LConn1
  Gear Constraint/RConn1 -- Hand/LConn3
  R1/RConn2 -- tA/RConn1
  R1/RConn3 -- tW/RConn1
  R2/RConn2 -- bA/RConn1
  R2/RConn3 -- bW/RConn1
  R3/RConn2 -- fA/RConn1
  R3/RConn3 -- fW/RConn1
  R4/RConn2 -- wA/RConn1
  R4/RConn3 -- wW/RConn1
  R5/RConn2 -- hA/RConn1
  R5/RConn3 -- hW/RConn1
  R7/RConn2 -- gA/RConn1
  R7/RConn3 -- gW/RConn1

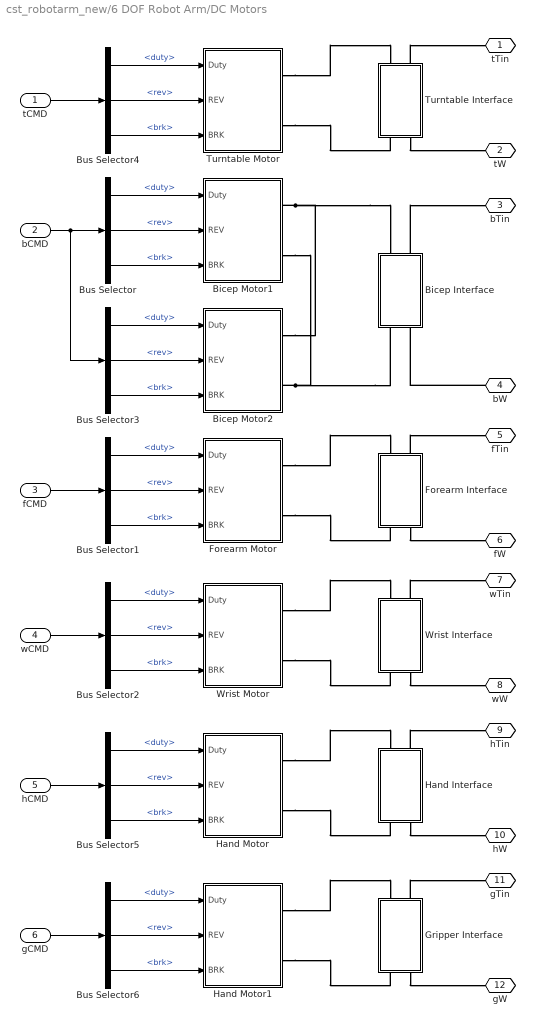
== system cst_robotarm_new/6 DOF Robot Arm/DC Motors ==
  tCMD : Inport
  bCMD : Inport  Port=2
  fCMD : Inport  Port=3
  wCMD : Inport  Port=4
  hCMD : Inport  Port=5
  gCMD : Inport  Port=6
  Bicep Interface : Subsystem
  Bicep Motor1 : Subsystem
      mask Display: image('Servo.jpg')
  Bicep Motor2 : Subsystem
      mask Display: image('Servo.jpg')
  Bus Selector{,1..6} (7 alike) : BusSelector  OutputSignals=duty,rev,brk
  Forearm Interface : Subsystem
  Forearm Motor : Subsystem
      mask Display: image('Servo.jpg')
  Gripper Interface : Subsystem
  Hand Interface : Subsystem
  Hand Motor : Subsystem
      mask Display: image('Servo.jpg')
  Hand Motor1 : Subsystem
      mask Display: image('Servo.jpg')
  Turntable Interface : Subsystem
  Turntable Motor : Subsystem
      mask Display: image('Servo.jpg')
  Wrist Interface : Subsystem
  Wrist Motor : Subsystem
      mask Display: image('Servo.jpg')
  tTin : PMIOPort  Side=Right
  tW : PMIOPort  Port=2  Side=Right
  bTin : PMIOPort  Port=3  Side=Right
  bW : PMIOPort  Port=4  Side=Right
  fTin : PMIOPort  Port=5  Side=Right
  fW : PMIOPort  Port=6  Side=Right
  wTin : PMIOPort  Port=7  Side=Right
  wW : PMIOPort  Port=8  Side=Right
  hTin : PMIOPort  Port=9  Side=Right
  hW : PMIOPort  Port=10  Side=Right
  gTin : PMIOPort  Port=11  Side=Right
  gW : PMIOPort  Port=12  Side=Right
  wires:
  bCMD/1 -> Bus Selector/1, Bus Selector3/1
  Bus Selector/1 -> Bicep Motor1/1(Duty)  "<duty>"
  Bus Selector/2 -> Bicep Motor1/2(REV)  "<rev>"
  Bus Selector/3 -> Bicep Motor1/3(BRK)  "<brk>"
  fCMD/1 -> Bus Selector1/1
  Bus Selector1/1 -> Forearm Motor/1(Duty)  "<duty>"
  Bus Selector1/2 -> Forearm Motor/2(REV)  "<rev>"
  Bus Selector1/3 -> Forearm Motor/3(BRK)  "<brk>"
  Bus Selector3/1 -> Bicep Motor2/1(Duty)  "<duty>"
  Bus Selector3/2 -> Bicep Motor2/2(REV)  "<rev>"
  Bus Selector3/3 -> Bicep Motor2/3(BRK)  "<brk>"
  wCMD/1 -> Bus Selector2/1
  Bus Selector2/1 -> Wrist Motor/1(Duty)  "<duty>"
  Bus Selector2/2 -> Wrist Motor/2(REV)  "<rev>"
  Bus Selector2/3 -> Wrist Motor/3(BRK)  "<brk>"
  tCMD/1 -> Bus Selector4/1
  Bus Selector4/1 -> Turntable Motor/1(Duty)  "<duty>"
  Bus Selector4/2 -> Turntable Motor/2(REV)  "<rev>"
  Bus Selector4/3 -> Turntable Motor/3(BRK)  "<brk>"
  hCMD/1 -> Bus Selector5/1
  Bus Selector5/1 -> Hand Motor/1(Duty)  "<duty>"
  Bus Selector5/2 -> Hand Motor/2(REV)  "<rev>"
  Bus Selector5/3 -> Hand Motor/3(BRK)  "<brk>"
  gCMD/1 -> Bus Selector6/1
  Bus Selector6/1 -> Hand Motor1/1(Duty)  "<duty>"
  Bus Selector6/2 -> Hand Motor1/2(REV)  "<rev>"
  Bus Selector6/3 -> Hand Motor1/3(BRK)  "<brk>"
  connections:
  Bicep Motor1/RConn1 -- Bicep Motor2/RConn1 -- Bicep Interface/LConn1
  Bicep Motor2/RConn2 -- Bicep Motor1/RConn2 -- Bicep Interface/RConn1
  Forearm Motor/RConn2 -- Forearm Interface/RConn1
  Forearm Motor/RConn1 -- Forearm Interface/LConn1
  Forearm Interface/RConn2 -- fW/RConn1
  Bicep Interface/LConn2 -- bTin/RConn1
  Forearm Interface/LConn2 -- fTin/RConn1
  bW/RConn1 -- Bicep Interface/RConn2
  Wrist Motor/RConn2 -- Wrist Interface/RConn1
  Wrist Interface/LConn2 -- wTin/RConn1
  Wrist Motor/RConn1 -- Wrist Interface/LConn1
  Wrist Interface/RConn2 -- wW/RConn1
  Turntable Interface/LConn2 -- tTin/RConn1
  Turntable Motor/RConn1 -- Turntable Interface/LConn1
  Turntable Motor/RConn2 -- Turntable Interface/RConn1
  Turntable Interface/RConn2 -- tW/RConn1
  Hand Interface/RConn2 -- hW/RConn1
  Hand Motor/RConn1 -- Hand Interface/LConn1
  Hand Interface/LConn2 -- hTin/RConn1
  Hand Motor/RConn2 -- Hand Interface/RConn1
  Hand Motor1/RConn2 -- Gripper Interface/RConn1
  Gripper Interface/RConn2 -- gW/RConn1
  Hand Motor1/RConn1 -- Gripper Interface/LConn1
  Gripper Interface/LConn2 -- gTin/RConn1

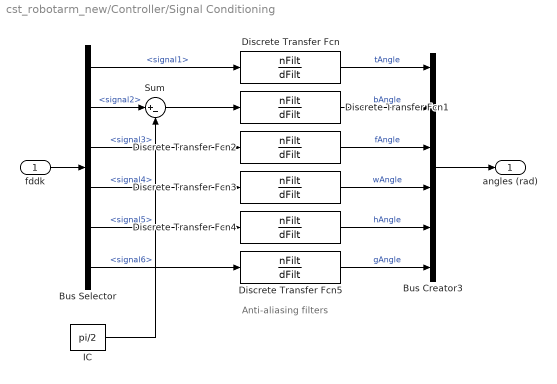
== system cst_robotarm_new/Controller/Signal Conditioning ==
  note: Anti-aliasing filters
  fddk : Inport
  Bus Creator3 : BusCreator  Inputs=6
  Bus Selector : BusSelector  OutputSignals=signal1,signal2,signal3,signal4,signal5,signal6
  Discrete Transfer Fcn{,1..5} (6 alike) : DiscreteTransferFcn  Numerator=nFilt  Denominator=dFilt  SampleTime=Ts
  IC : Constant  Value=pi/2
  Sum : Sum  Inputs=|+-
  angles (rad) : Outport  VectorParamsAs1DForOutWhenUnconnected=off
  wires:
  Discrete Transfer Fcn1/1 -> Bus Creator3/2  "bAngle"
  Discrete Transfer Fcn/1 -> Bus Creator3/1  "tAngle"
  fddk/1 -> Bus Selector/1
  Bus Selector/1 -> Discrete Transfer Fcn/1  "<signal1>"
  Bus Selector/4 -> Discrete Transfer Fcn3/1  "<signal4>"
  Bus Selector/3 -> Discrete Transfer Fcn2/1  "<signal3>"
  Discrete Transfer Fcn2/1 -> Bus Creator3/3  "fAngle"
  Discrete Transfer Fcn3/1 -> Bus Creator3/4  "wAngle"
  Bus Creator3/1 -> angles (rad)/1
  Discrete Transfer Fcn4/1 -> Bus Creator3/5  "hAngle"
  Discrete Transfer Fcn5/1 -> Bus Creator3/6  "gAngle"
  Bus Selector/5 -> Discrete Transfer Fcn4/1  "<signal5>"
  Bus Selector/6 -> Discrete Transfer Fcn5/1  "<signal6>"
  Bus Selector/2 -> Sum/1  "<signal2>"
  Sum/1 -> Discrete Transfer Fcn1/1
  IC/1 -> Sum/2

== system cst_robotarm_new/Controller/bicepCMD ==
  Vcmd : Inport
  Vbrk : Inport  Port=2
  Abs : Abs
  Fcn : Fcn  Expr=u(1)<0
  Gain : Gain  Gain=5
  "[0...5]" : Saturate  UpperLimit=5  LowerLimit=0
  "[0...5] " : Saturate  UpperLimit=5  LowerLimit=0
  Duty : Outport  VectorParamsAs1DForOutWhenUnconnected=off
  REV : Outport  Port=2  VectorParamsAs1DForOutWhenUnconnected=off
  BRK : Outport  Port=3  VectorParamsAs1DForOutWhenUnconnected=off
  wires:
  Gain/1 -> REV/1
  "[0...5]"/1 -> Duty/1
  Fcn/1 -> Gain/1
  Abs/1 -> "[0...5]"/1
  Vcmd/1 -> Abs/1, Fcn/1
  Vbrk/1 -> "[0...5] "/1
  "[0...5] "/1 -> BRK/1

== system cst_robotarm_new/Controller/bicepPID ==
  bref : Inport
  bangle : Inport  Port=2
  Derivative : Derivative
  Gd2 : Gain  Gain=10
  Gi2 : Gain  Gain=17.40
  Gp2 : Gain  Gain=19.28
  Integrator : Integrator
  Sum : Sum  Inputs=|+-
  Sum2 : Sum  Inputs=+++
  bcmd : Outport
  wires:
  Derivative/1 -> Gd2/1
  Integrator/1 -> Gi2/1
  Gd2/1 -> Sum2/3  "Kd2"
  Gi2/1 -> Sum2/1  "Ki2"
  Gp2/1 -> Sum2/2  "Kp2"
  Sum2/1 -> bcmd/1
  Sum/1 -> Integrator/1, Derivative/1, Gp2/1
  bref/1 -> Sum/1
  bangle/1 -> Sum/2

== system cst_robotarm_new/Controller/forearPID ==
  fref : Inport
  fangle : Inport  Port=2
  Derivative : Derivative
  Gd3 : Gain  Gain=10
  Gi3 : Gain  Gain=12.40
  Gp3 : Gain  Gain=11.69
  Integrator : Integrator
  Sum : Sum  Inputs=|+-
  Sum2 : Sum  Inputs=+++
  fcmd : Outport
  wires:
  Derivative/1 -> Gd3/1
  Integrator/1 -> Gi3/1
  Gd3/1 -> Sum2/3  "Kd3"
  Gi3/1 -> Sum2/1  "Ki3"
  Gp3/1 -> Sum2/2  "Kp3"
  Sum2/1 -> fcmd/1
  Sum/1 -> Derivative/1, Integrator/1, Gp3/1
  fref/1 -> Sum/1
  fangle/1 -> Sum/2

== system cst_robotarm_new/Controller/forearmCMD ==
  Vcmd : Inport
  Vbrk : Inport  Port=2
  Abs : Abs
  Fcn : Fcn  Expr=u(1)<0
  Gain : Gain  Gain=5
  "[0...5]" : Saturate  UpperLimit=5  LowerLimit=0
  "[0...5] " : Saturate  UpperLimit=5  LowerLimit=0
  Duty : Outport  VectorParamsAs1DForOutWhenUnconnected=off
  REV : Outport  Port=2  VectorParamsAs1DForOutWhenUnconnected=off
  BRK : Outport  Port=3  VectorParamsAs1DForOutWhenUnconnected=off
  wires:
  "[0...5] "/1 -> BRK/1
  Vbrk/1 -> "[0...5] "/1
  Vcmd/1 -> Fcn/1, Abs/1
  Abs/1 -> "[0...5]"/1
  Fcn/1 -> Gain/1
  "[0...5]"/1 -> Duty/1
  Gain/1 -> REV/1

== system cst_robotarm_new/Controller/gripperCMD ==
  Vcmd : Inport
  Vbrk : Inport  Port=2
  Abs : Abs
  Fcn : Fcn  Expr=u(1)<0
  Gain : Gain  Gain=5
  "[0...5]" : Saturate  UpperLimit=5  LowerLimit=0
  "[0...5] " : Saturate  UpperLimit=5  LowerLimit=0
  Duty : Outport  VectorParamsAs1DForOutWhenUnconnected=off
  REV : Outport  Port=2  VectorParamsAs1DForOutWhenUnconnected=off
  BRK : Outport  Port=3  VectorParamsAs1DForOutWhenUnconnected=off
  wires:
  "[0...5] "/1 -> BRK/1
  Vbrk/1 -> "[0...5] "/1
  Vcmd/1 -> Fcn/1, Abs/1
  Abs/1 -> "[0...5]"/1
  Fcn/1 -> Gain/1
  "[0...5]"/1 -> Duty/1
  Gain/1 -> REV/1

== system cst_robotarm_new/Controller/gripperPID ==
  gref : Inport
  gangle : Inport  Port=2
  Derivative : Derivative
  Gd6 : Gain  Gain=10
  Gi6 : Gain  Gain=12.06
  Gp6 : Gain  Gain=10.84
  Integrator : Integrator
  Sum : Sum  Inputs=|+-
  Sum2 : Sum  Inputs=+++
  gcmd : Outport
  wires:
  Derivative/1 -> Gd6/1
  Integrator/1 -> Gi6/1
  Gd6/1 -> Sum2/3  "Kd6"
  Gi6/1 -> Sum2/1  "Ki6"
  Gp6/1 -> Sum2/2  "Kp6"
  Sum2/1 -> gcmd/1
  Sum/1 -> Integrator/1, Derivative/1, Gp6/1
  gref/1 -> Sum/1
  gangle/1 -> Sum/2

== system cst_robotarm_new/Controller/handCMD ==
  Vcmd : Inport
  Vbrk : Inport  Port=2
  Abs : Abs
  Fcn : Fcn  Expr=u(1)<0
  Gain : Gain  Gain=5
  "[0...5]" : Saturate  UpperLimit=5  LowerLimit=0
  "[0...5] " : Saturate  UpperLimit=5  LowerLimit=0
  Duty : Outport  VectorParamsAs1DForOutWhenUnconnected=off
  REV : Outport  Port=2  VectorParamsAs1DForOutWhenUnconnected=off
  BRK : Outport  Port=3  VectorParamsAs1DForOutWhenUnconnected=off
  wires:
  Gain/1 -> REV/1
  "[0...5]"/1 -> Duty/1
  Fcn/1 -> Gain/1
  Abs/1 -> "[0...5]"/1
  Vcmd/1 -> Abs/1, Fcn/1
  Vbrk/1 -> "[0...5] "/1
  "[0...5] "/1 -> BRK/1

== system cst_robotarm_new/Controller/handPID ==
  <fREF> : Inport
  <hAngle> : Inport  Port=2
  Derivative : Derivative
  Gd5 : Gain  Gain=10
  Gi5 : Gain
  Gp5 : Gain  Gain=11.18
  Integrator : Integrator
  Sum : Sum  Inputs=|+-
  Sum2 : Sum  Inputs=+++
  hCMD : Outport
  wires:
  Sum2/1 -> hCMD/1  "hCMD"
  Derivative/1 -> Gd5/1
  Sum/1 -> Integrator/1, Derivative/1, Gp5/1
  Gd5/1 -> Sum2/3  "Kd5"
  <hAngle>/1 -> Sum/2
  Integrator/1 -> Gi5/1
  <fREF>/1 -> Sum/1
  Gp5/1 -> Sum2/2  "Kp5"
  Gi5/1 -> Sum2/1  "Ki5"

== system cst_robotarm_new/Controller/turntableCMD ==
  Vcmd : Inport
  Vbrk : Inport  Port=2
  Abs : Abs
  Fcn : Fcn  Expr=u(1)<0
  Gain : Gain  Gain=5
  "[0...5]" : Saturate  UpperLimit=5  LowerLimit=0
  "[0...5] " : Saturate  UpperLimit=5  LowerLimit=0
  Duty : Outport  VectorParamsAs1DForOutWhenUnconnected=off
  REV : Outport  Port=2  VectorParamsAs1DForOutWhenUnconnected=off
  BRK : Outport  Port=3  VectorParamsAs1DForOutWhenUnconnected=off
  wires:
  "[0...5] "/1 -> BRK/1
  Vbrk/1 -> "[0...5] "/1
  Vcmd/1 -> Fcn/1, Abs/1
  Abs/1 -> "[0...5]"/1
  Fcn/1 -> Gain/1
  "[0...5]"/1 -> Duty/1
  Gain/1 -> REV/1

== system cst_robotarm_new/Controller/turntablePID ==
  tref : Inport
  tangle : Inport  Port=2
  Derivative : Derivative
  Gd1 : Gain  Gain=10
  Gi1 : Gain  Gain=11.76
  Gp1 : Gain  Gain=10.19
  Integrator : Integrator
  Sum : Sum  Inputs=|+-
  Sum2 : Sum  Inputs=+++
  tcmd : Outport
  wires:
  Derivative/1 -> Gd1/1
  Integrator/1 -> Gi1/1
  Gd1/1 -> Sum2/3  "Kd1"
  Gi1/1 -> Sum2/1  "Ki1"
  Gp1/1 -> Sum2/2  "Kp1"
  Sum2/1 -> tcmd/1
  Sum/1 -> Integrator/1, Derivative/1, Gp1/1
  tref/1 -> Sum/1
  tangle/1 -> Sum/2

== system cst_robotarm_new/Controller/wristCMD ==
  Vcmd : Inport
  Vbrk : Inport  Port=2
  Abs : Abs
  Fcn : Fcn  Expr=u(1)<0
  Gain : Gain  Gain=5
  "[0...5]" : Saturate  UpperLimit=5  LowerLimit=0
  "[0...5] " : Saturate  UpperLimit=5  LowerLimit=0
  Duty : Outport  VectorParamsAs1DForOutWhenUnconnected=off
  REV : Outport  Port=2  VectorParamsAs1DForOutWhenUnconnected=off
  BRK : Outport  Port=3  VectorParamsAs1DForOutWhenUnconnected=off
  wires:
  "[0...5] "/1 -> BRK/1
  Vbrk/1 -> "[0...5] "/1
  Vcmd/1 -> Fcn/1, Abs/1
  Abs/1 -> "[0...5]"/1
  Fcn/1 -> Gain/1
  "[0...5]"/1 -> Duty/1
  Gain/1 -> REV/1

== system cst_robotarm_new/Controller/wristPID ==
  wref : Inport
  wangle : Inport  Port=2
  Derivative : Derivative
  Gd4 : Gain  Gain=10
  Gi4 : Gain  Gain=11.09
  Gp4 : Gain  Gain=9.18
  Integrator : Integrator
  Sum : Sum  Inputs=|+-
  Sum2 : Sum  Inputs=+++
  wcmd : Outport
  wires:
  Derivative/1 -> Gd4/1
  Integrator/1 -> Gi4/1
  Gd4/1 -> Sum2/3  "Kd4"
  Gi4/1 -> Sum2/1  "Ki4"
  Gp4/1 -> Sum2/2  "Kp4"
  Sum2/1 -> wcmd/1
  Sum/1 -> Integrator/1, Derivative/1, Gp4/1
  wref/1 -> Sum/1
  wangle/1 -> Sum/2

== system cst_robotarm_new/6 DOF Robot Arm/6 DOF Robot Arm Mechanics/Base ==
  ReferenceFrame : sm_lib/Frames and Transforms/Reference Frame
  Solid : sm_lib/Body Elements/File Solid  ExtGeomFileName=BaseRef_Default_sldprt.STL  UnitType=Custom  ExtGeomFileUnits=in  StepReaderType=HEX  ExportConvexHullGeometry=off  InertiaType=Custom  Mass=0.0048917083782427382  MassUnits=kg  CenterOfMass=[-1.7039170891361811e-10 0.2623949674376988 1.6125651751179532e-08]  CenterOfMassUnits=in  MomentsOfInertia=[0.0003243123013680548 0.00029766954875355879 0.00032242565061571212]  MomentsOfInertiaUnits=kg*in^2  ProductsOfInertia=[-6.4526471956204744e-12 2.3575705931561807e-11 0]  ProductsOfInertiaUnits=kg*in^2  BasedOnType=Density  Density=1000  DensityUnits=kg/(m^3)  DoExposeReferenceFrame=on  SerializedFrames=<Frames/>  GraphicType=FromGeometry  MarkerShape=Sphere  MarkerSize=10  MarkerSizeUnits=m  GraphicVisPropType=SimpleVisualProperties  GraphicDiffuseColor=[0.4 0.4 0.4]  GraphicSpecularColor=[0.5 0.5 0.5 1.0]  GraphicAmbientColor=[0.15 0.15 0.15 1.0]  GraphicEmissiveColor=[0.0 0.0 0.0 1.0]  GraphicShininess=75  GraphicOpacity=1
  Transform : sm_lib/Frames and Transforms/Rigid Transform  TranslationMethod=Cartesian  TranslationStandardOffset=0  TranslationLengthUnit=mm  TranslationStandardAxis=+Z  TranslationCartesianOffset=[0 0 0]  TranslationROffset=0  TranslationROffsetUnits=m  TranslationZOffset=0  TranslationZOffsetUnits=m  TranslationThetaOffset=0  TranslationThetaOffsetUnits=deg  RotationMethod=ArbitraryAxis  RotationAngleUnits=rad  RotationStandardAxis=+Z  RotationAngle=2.0943951023931953  RotationArbitraryAxis=[0.57735026918962584 -0.57735026918962584 0.57735026918962584]  FollAlignAxisA=+X  BaseAlignAxisA=+Y  FollAlignAxisB=+Y  BaseAlignAxisB=+Z  RotationSequenceAxes=FollowerAxes  RotationSequence=XYX  RotationSequenceAngles=[0 0 0]  RotationSequenceAnglesUnits=deg  RotationMatrix=[1 0 0; 0 1 0; 0 0 1]
  Transform1 : sm_lib/Frames and Transforms/Rigid Transform  TranslationMethod=None  TranslationStandardOffset=0  TranslationLengthUnit=mm  TranslationStandardAxis=+Z  TranslationCartesianOffset=[0 0 0]  TranslationROffset=0  TranslationROffsetUnits=m  TranslationZOffset=0  TranslationZOffsetUnits=m  TranslationThetaOffset=0  TranslationThetaOffsetUnits=deg  RotationMethod=StandardAxis  RotationAngleUnits=deg  RotationStandardAxis=+X  RotationAngle=180  RotationArbitraryAxis=[0.57735026918962584 -0.57735026918962584 0.57735026918962584]  FollAlignAxisA=+X  BaseAlignAxisA=+Y  FollAlignAxisB=+Y  BaseAlignAxisB=+Z  RotationSequenceAxes=FollowerAxes  RotationSequence=XYX  RotationSequenceAngles=[0 0 0]  RotationSequenceAnglesUnits=deg  RotationMatrix=[1 0 0; 0 1 0; 0 0 1]
  F1 : PMIOPort  Side=Left
  F : PMIOPort  Port=2  Side=Right
  connections:
  ReferenceFrame/RConn1 -- Transform/LConn1 -- Solid/RConn1 -- F1/RConn1
  Transform1/RConn1 -- F/RConn1
  Transform/RConn1 -- Transform1/LConn1
